simulink model "Ex_10_Open_Loop_With_Disturbance_Observer"  (Simulink 9.0)
settings: Solver=ode3  StartTime=0.0  StopTime=t_max  FixedStep=jointObj.Ts  RelTol=1e-3
values from neighbouring files (symbols this model uses):
  t_max = f_max    (= 100)    [Ex_00_example_config.m]
libraries: simulink x1, cjt_library_observers x1, cjt_library_models x1
settings Model: Creator=joern  LastModifiedBy=J�rn
settings DebuggingCC: UnderspecifiedInitializationDetection=Simplified  MergeDetectMultiDrivingBlocksExec=error  SolverPrmCheckMsg=warning
settings GRTTargetCC: GeneratePreprocessorConditionals=Disable all
settings ConfigComp: CovSFcnEnable=off

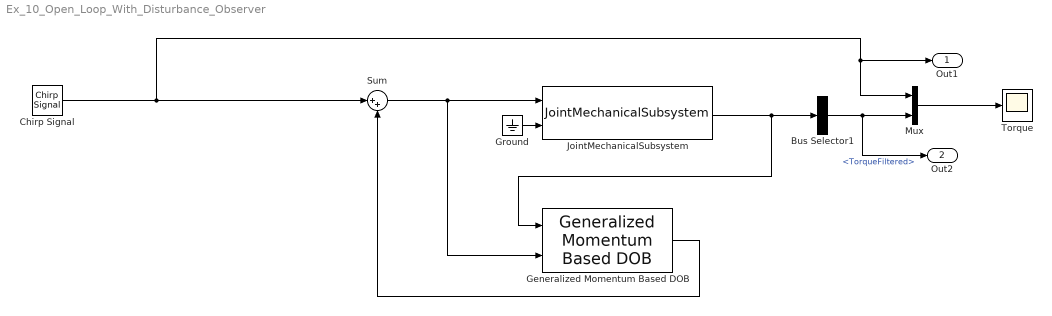
== system Ex_10_Open_Loop_With_Disturbance_Observer ==
  Bus Selector1 : BusSelector  OutputSignals=TorqueFiltered
  Chirp Signal : simulink/Sources/Chirp Signal  f1=f_min  T=t_max  f2=f_max
  Generalized Momentum Based DOB : cjt_library_observers/Observers/Generalized Momentum Based DOB  jointObj=jointObj  L=2*pi*25
  Ground : Ground
  JointMechanicalSubsystem : cjt_library_models/Joint models/JointMechanicalSubsystem  jointObj=jointObj  fc_vel=499  fc_torque=499  input_delay=1  output_delay=1  quantize=on  quantize_bits=19  input_noise_enabled=off  output_noise_enabled=off  var_u=0.12^2  var_y=1.8e-10
  Mux : Mux  Inputs=2
  Sum : Sum  Inputs=|++
  Torque : Scope
  Out1 : Outport  SignalName=Reference
  Out2 : Outport  Port=2  SignalName=Response
  wires:
  Mux/1 -> Torque/1
  Ground/1 -> JointMechanicalSubsystem/2
  JointMechanicalSubsystem/1 -> Generalized Momentum Based DOB/1, Bus Selector1/1
  Sum/1 -> Generalized Momentum Based DOB/2, JointMechanicalSubsystem/1
  Chirp Signal/1 -> Sum/1, Out1/1, Mux/1
  Bus Selector1/1 -> Out2/1, Mux/2  "<TorqueFiltered>"
  Generalized Momentum Based DOB/1 -> Sum/2
